simulink model "PMSMControlWithLPF"  (R2022b)
settings: Solver=FixedStepAuto  StartTime=0.0  StopTime=10  RelTol=1e-3
values from neighbouring files (symbols this model uses):
  Ls = 0.01    [Parameters.m]
  R = 1    [Parameters.m]
libraries: simulink x1
settings Model: Creator=ahmed  LastModifiedBy=ahmed

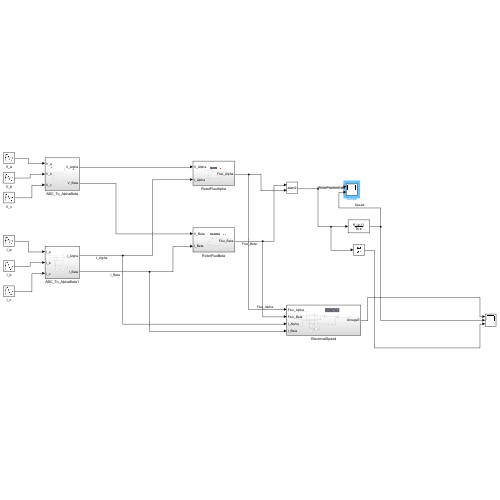
[thumbnail: Simulink's stored preview of the top-level diagram]
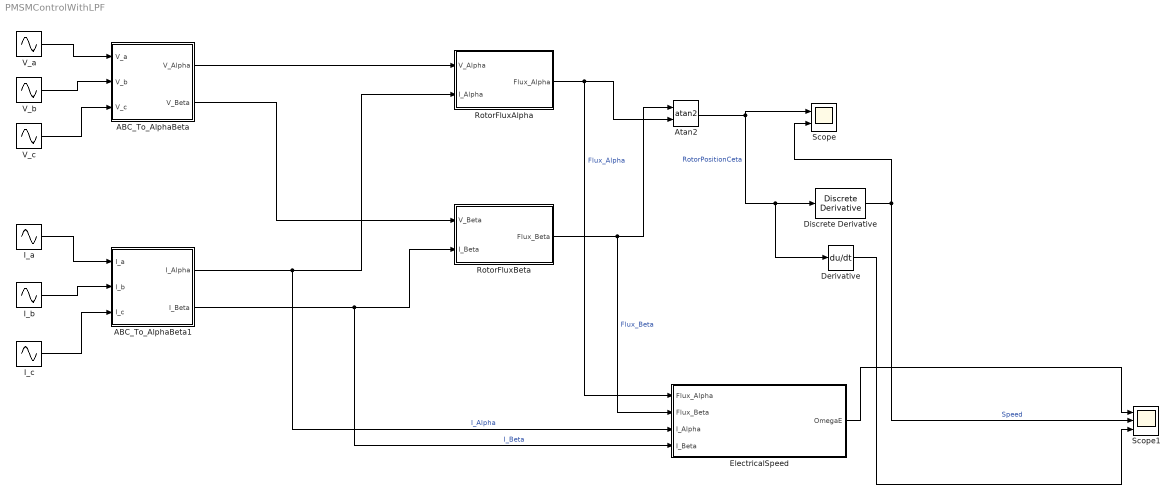
== system PMSMControlWithLPF ==
  ABC_To_AlphaBeta : Subsystem
  ABC_To_AlphaBeta1 : Subsystem
  Atan2 : Trigonometry  Operator=atan2
  Derivative : Derivative
  Discrete Derivative : simulink/Discrete/Discrete Derivative  gainval=1.0  ICPrevScaledInput=0.0  OutMin=[]  OutMax=[]  OutDataType=fixdt(1, 16)  OutScaling=2^-10  DoSatur=off
  ElectricalSpeed : Subsystem
  I_a : Sin  Amplitude=2  Frequency=300  SampleTime=0
  I_b : Sin  Amplitude=2  Frequency=300  Phase=-120 * (pi/180)  SampleTime=0
  I_c : Sin  Amplitude=2  Frequency=300  Phase=120 * (pi/180)  SampleTime=0
  RotorFluxAlpha : Subsystem
  RotorFluxBeta : Subsystem
  Scope : Scope  NumInputPorts=2
  Scope1 : Scope  NumInputPorts=3
  V_a : Sin  Amplitude=12  Frequency=300  SampleTime=0
  V_b : Sin  Amplitude=12  Frequency=300  Phase=-120 * (pi/180)  SampleTime=0
  V_c : Sin  Amplitude=12  Frequency=300  Phase=120 * (pi/180)  SampleTime=0
  wires:
  V_a/1 -> ABC_To_AlphaBeta/1(V_a)
  V_b/1 -> ABC_To_AlphaBeta/2(V_b)
  V_c/1 -> ABC_To_AlphaBeta/3(V_c)
  I_c/1 -> ABC_To_AlphaBeta1/3(I_c)
  I_b/1 -> ABC_To_AlphaBeta1/2(I_b)
  I_a/1 -> ABC_To_AlphaBeta1/1(I_a)
  ABC_To_AlphaBeta/1(V_Alpha) -> RotorFluxAlpha/1(V_Alpha)
  ABC_To_AlphaBeta1/1(I_Alpha) -> ElectricalSpeed/3(I_Alpha), RotorFluxAlpha/2(I_Alpha)  "I_Alpha"
  ABC_To_AlphaBeta/2(V_Beta) -> RotorFluxBeta/1(V_Beta)
  ABC_To_AlphaBeta1/2(I_Beta) -> ElectricalSpeed/4(I_Beta), RotorFluxBeta/2(I_Beta)  "I_Beta"
  RotorFluxAlpha/1(Flux_Alpha) -> ElectricalSpeed/1(Flux_Alpha), Atan2/2  "Flux_Alpha"
  RotorFluxBeta/1(Flux_Beta) -> ElectricalSpeed/2(Flux_Beta), Atan2/1  "Flux_Beta"
  Atan2/1 -> Derivative/1, Discrete Derivative/1, Scope/1  "RotorPositionCeta"
  ElectricalSpeed/1(OmegaE) -> Scope1/1
  Discrete Derivative/1 -> Scope/2, Scope1/2  "Speed"
  Derivative/1 -> Scope1/3

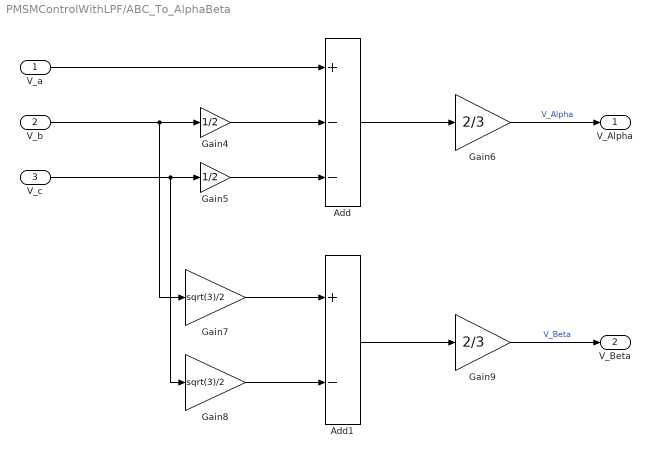
== system PMSMControlWithLPF/ABC_To_AlphaBeta ==
  V_a : Inport
  V_b : Inport  Port=2
  V_c : Inport  Port=3
  Add : Sum  Inputs=+--
  Add1 : Sum  Inputs=+-
  Gain4 : Gain  Gain=1/2
  Gain5 : Gain  Gain=1/2
  Gain6 : Gain  Gain=2/3
  Gain7 : Gain  Gain=sqrt(3)/2
  Gain8 : Gain  Gain=sqrt(3)/2
  Gain9 : Gain  Gain=2/3
  V_Alpha : Outport
  V_Beta : Outport  Port=2
  wires:
  Add1/1 -> Gain9/1
  Gain4/1 -> Add/2
  V_c/1 -> Gain8/1, Gain5/1
  Gain5/1 -> Add/3
  Add/1 -> Gain6/1
  Gain7/1 -> Add1/1
  Gain8/1 -> Add1/2
  Gain9/1 -> V_Beta/1  "V_Beta"
  V_b/1 -> Gain7/1, Gain4/1
  Gain6/1 -> V_Alpha/1  "V_Alpha"
  V_a/1 -> Add/1

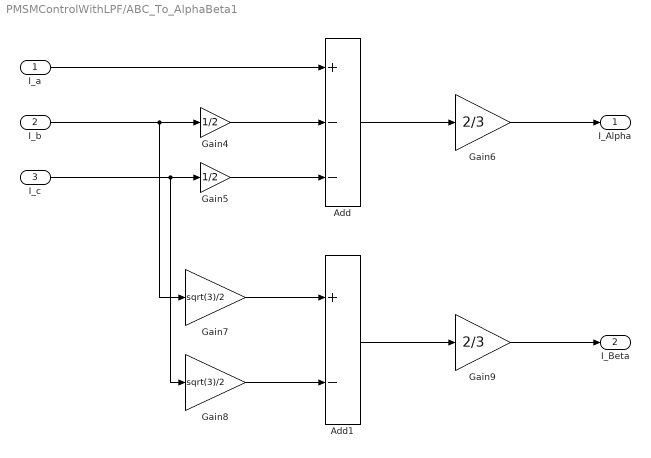
== system PMSMControlWithLPF/ABC_To_AlphaBeta1 ==
  I_a : Inport
  I_b : Inport  Port=2
  I_c : Inport  Port=3
  Add : Sum  Inputs=+--
  Add1 : Sum  Inputs=+-
  Gain4 : Gain  Gain=1/2
  Gain5 : Gain  Gain=1/2
  Gain6 : Gain  Gain=2/3
  Gain7 : Gain  Gain=sqrt(3)/2
  Gain8 : Gain  Gain=sqrt(3)/2
  Gain9 : Gain  Gain=2/3
  I_Alpha : Outport
  I_Beta : Outport  Port=2
  wires:
  Add1/1 -> Gain9/1
  Gain4/1 -> Add/2
  I_c/1 -> Gain8/1, Gain5/1
  Gain5/1 -> Add/3
  Add/1 -> Gain6/1
  Gain7/1 -> Add1/1
  Gain8/1 -> Add1/2
  Gain9/1 -> I_Beta/1
  I_b/1 -> Gain7/1, Gain4/1
  Gain6/1 -> I_Alpha/1
  I_a/1 -> Add/1

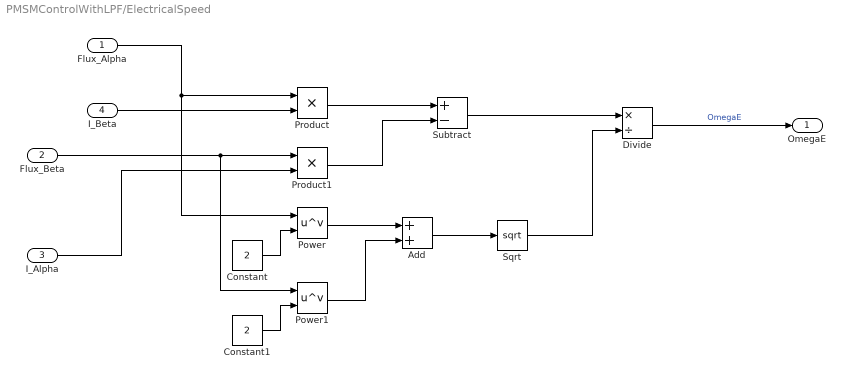
== system PMSMControlWithLPF/ElectricalSpeed ==
  Flux_Alpha : Inport
  Flux_Beta : Inport  Port=2
  I_Alpha : Inport  Port=3
  I_Beta : Inport  Port=4
  Add : Sum
  Constant : Constant  Value=2
  Constant1 : Constant  Value=2
  Divide : Product  Inputs=*/
  Power : Math  Operator=pow
  Power1 : Math  Operator=pow
  Product : Product
  Product1 : Product
  Sqrt : Sqrt
  Subtract : Sum  Inputs=+-
  OmegaE : Outport
  wires:
  Flux_Alpha/1 -> Power/1, Product/1
  Power1/1 -> Add/2
  Subtract/1 -> Divide/1
  Constant1/1 -> Power1/2
  Product1/1 -> Subtract/2
  Power/1 -> Add/1
  Sqrt/1 -> Divide/2
  I_Beta/1 -> Product/2
  Flux_Beta/1 -> Product1/1, Power1/1
  Constant/1 -> Power/2
  Product/1 -> Subtract/1
  Add/1 -> Sqrt/1
  Divide/1 -> OmegaE/1  "OmegaE"
  I_Alpha/1 -> Product1/2

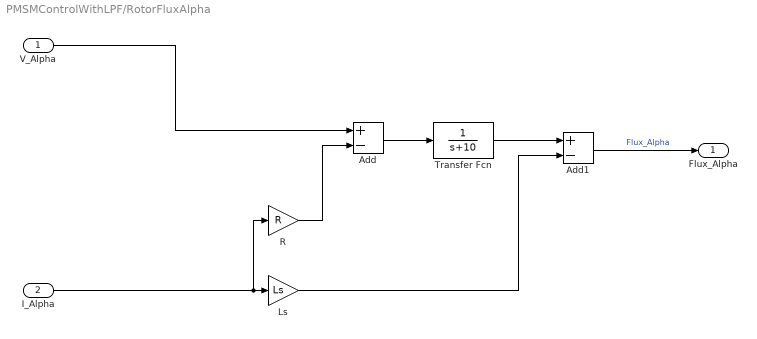
== system PMSMControlWithLPF/RotorFluxAlpha ==
  V_Alpha : Inport
  I_Alpha : Inport  Port=2
  Add : Sum  Inputs=+-
  Add1 : Sum  Inputs=+-
  Ls : Gain  Gain=Ls
  R : Gain  Gain=R
  Transfer Fcn : TransferFcn  Denominator=[1 10]
  Flux_Alpha : Outport
  wires:
  I_Alpha/1 -> R/1, Ls/1
  V_Alpha/1 -> Add/1
  Ls/1 -> Add1/2
  Add1/1 -> Flux_Alpha/1  "Flux_Alpha"
  R/1 -> Add/2
  Add/1 -> Transfer Fcn/1
  Transfer Fcn/1 -> Add1/1

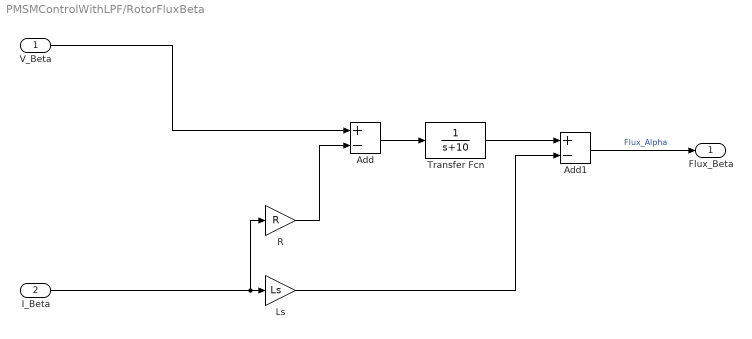
== system PMSMControlWithLPF/RotorFluxBeta ==
  V_Beta : Inport
  I_Beta : Inport  Port=2
  Add : Sum  Inputs=+-
  Add1 : Sum  Inputs=+-
  Ls : Gain  Gain=Ls
  R : Gain  Gain=R
  Transfer Fcn : TransferFcn  Denominator=[1 10]
  Flux_Beta : Outport
  wires:
  R/1 -> Add/2
  Transfer Fcn/1 -> Add1/1
  Add1/1 -> Flux_Beta/1  "Flux_Alpha"
  Ls/1 -> Add1/2
  V_Beta/1 -> Add/1
  Add/1 -> Transfer Fcn/1
  I_Beta/1 -> Ls/1, R/1
